simulink model "TRAS_DevDriv"  (Simulink 8.1)
settings: Solver=ode5  SolverMode=SingleTasking  StartTime=0.0  StopTime=999999  FixedStep=0.01  RelTol=1e-3  AbsTol=1e-6
undefined symbols (not defined in the file): rtdac4pcibaseaddress
settings Model: Creator=jims  LastModifiedBy=inteco  SimulationMode=external  ExtModeTrigDuration=12000
settings DataIOCC: ExternalInput=[]  InitialState=[]  LimitDataPoints=off  MaxDataPoints=5000  SaveOutput=off  SaveTime=off  SignalLoggingName=sigsOut
settings OptimizationCC: BooleanDataType=off  InitFltsAndDblsToZero=on
settings DebuggingCC: SaveWithParameterizedLinksMsg=none  SignalResolutionControl=TryResolveAllWithWarning  SolverPrmCheckMsg=none  MultiTaskDSMMsg=warning  MultiTaskCondExecSysMsg=none  IntegerOverflowMsg=none  StrictBusMsg=None
settings HardwareCC: ProdIntDivRoundTo=Zero  ProdEndianess=LittleEndian  ProdHWDeviceType=Generic->32-bit x86 compatible
settings RTWCC: SystemTargetFile=rtwin.tlc  TemplateMakefile=rtwin.tmf  Description=Real-Time Windows Target  ProcessScript=rtwin_make_rtw_hook  IncludeERTFirstTime=on  RTWCompilerOptimization=On
settings CodeAppCC: MaxIdLength=95
settings RTWinTargetCC: TargetLibSuffix=_rtwin.lib  TargetPreCompLibLocation=E:\apps_W32\MATLAB\R2013a\toolbox\rtw\targets\rtwin\lib\win32  CodeReplacementLibrary=ANSI_C  RTWinDir=E:/apps_W32/MATLAB/R2013a/toolbox/rtw/targets/rtwin  TargetArch=win32

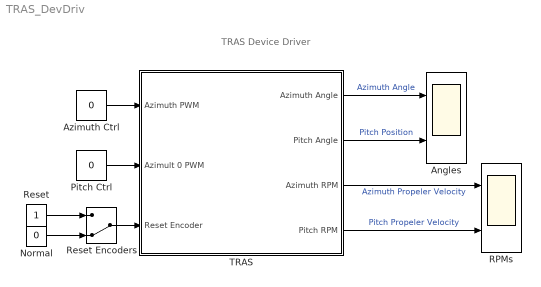
== system TRAS_DevDriv ==
  note: TRAS Device Driver
  Angles : Scope  NumInputPorts=2
      settings: TimeRange=30  YMin=-0.02~-0.1  YMax=0.0025~1  SaveName=SD1  MaxDataPoints=12000
  Azimuth Ctrl : Constant  Value=0
  Normal : Constant  Value=0
  Pitch Ctrl : Constant  Value=0
  RPMs : Scope  NumInputPorts=2
      settings: TimeRange=30  YMin=-20~-400  YMax=0~500  SaveName=SD  MaxDataPoints=12000
  Reset : Constant
  Reset Encoders : ManualSwitch  CurrentSetting=0
  TRAS : Subsystem  mask{BaseAddress=rtdac4pcibaseaddress, T0=0.01}
      mask prompts: BaseAddress "Base Address:"; T0 "Sampling Period:"
      mask Display: image(imread('TRAS.JPG'))
  wires:
  TRAS/1(Azimuth Angle) -> Angles/1  "Azimuth Angle"
  TRAS/2(Pitch Angle) -> Angles/2  "Pitch Position"
  Azimuth Ctrl/1 -> TRAS/1(Azimuth PWM)
  Pitch Ctrl/1 -> TRAS/2(Azimult 0 PWM)
  TRAS/3(Azimuth RPM) -> RPMs/1  "Azimuth Propeler Velocity"
  TRAS/4(Pitch RPM) -> RPMs/2  "Pitch Propeler Velocity"
  Normal/1 -> Reset Encoders/2
  Reset/1 -> Reset Encoders/1
  Reset Encoders/1 -> TRAS/3(Reset Encoder)

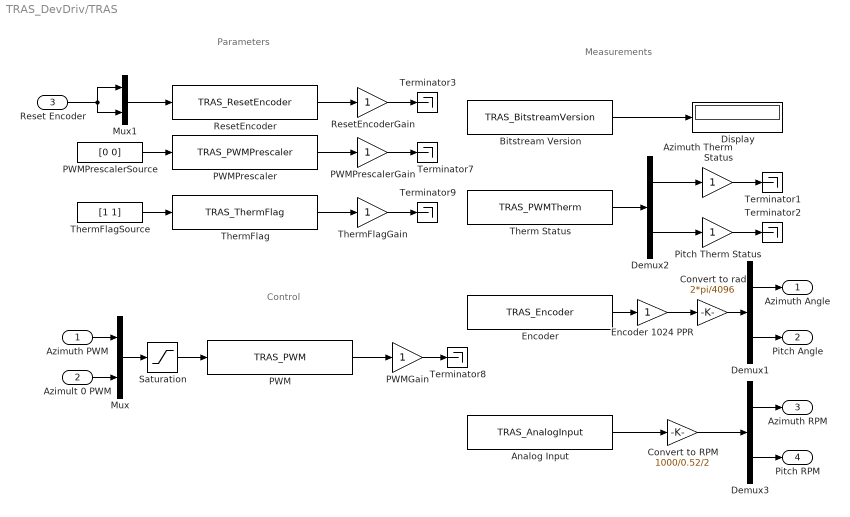
== system TRAS_DevDriv/TRAS ==
  note: Measurements
  note: Control
  note: Parameters
  Azimuth PWM : Inport
  Azimult 0 PWM : Inport  Port=2
  Reset Encoder : Inport  Port=3
  Analog Input : S-Function  FunctionName=TRAS_AnalogInput  Parameters=BaseAddress, [1 0], [1 1], T0  EnableBusSupport=off
  Azimuth Therm Status : Gain  SaturateOnIntegerOverflow=on  OutDataTypeStr=Inherit: Same as input  ParamDataTypeStr=Inherit: Same as input
  Bitstream Version : S-Function  FunctionName=TRAS_BitstreamVersion  Parameters=BaseAddress, T0  EnableBusSupport=off
  Convert to RPM : Gain  Gain=1000/0.52/2  SaturateOnIntegerOverflow=on  OutDataTypeStr=Inherit: Same as input  ParamDataTypeStr=Inherit: Same as input
  Convert to rad : Gain  Gain=2*pi/4096  SaturateOnIntegerOverflow=on  OutDataTypeStr=Inherit: Same as input  ParamDataTypeStr=Inherit: Same as input
  Demux1 : Demux  Outputs=2
  Demux2 : Demux  Outputs=2
  Demux3 : Demux  Outputs=2
  Display : Display
  Encoder : S-Function  FunctionName=TRAS_Encoder  Parameters=BaseAddress, T0  EnableBusSupport=off
  Encoder 1024 PPR : Gain  SaturateOnIntegerOverflow=on  OutDataTypeStr=Inherit: Same as input  ParamDataTypeStr=Inherit: Same as input
  Mux : Mux  Inputs=2
  Mux1 : Mux  Inputs=2
  PWM : S-Function  FunctionName=TRAS_PWM  Parameters=BaseAddress, T0  EnableBusSupport=off
  PWMGain : Gain  SaturateOnIntegerOverflow=on  OutDataTypeStr=Inherit: Same as input  ParamDataTypeStr=Inherit: Same as input
  PWMPrescaler : S-Function  FunctionName=TRAS_PWMPrescaler  Parameters=BaseAddress, T0  EnableBusSupport=off
  PWMPrescalerGain : Gain  SaturateOnIntegerOverflow=on  OutDataTypeStr=Inherit: Same as input  ParamDataTypeStr=Inherit: Same as input
  PWMPrescalerSource : Constant  Value=[0 0]
  Pitch Therm Status : Gain  SaturateOnIntegerOverflow=on  OutDataTypeStr=Inherit: Same as input  ParamDataTypeStr=Inherit: Same as input
  ResetEncoder : S-Function  FunctionName=TRAS_ResetEncoder  Parameters=BaseAddress, T0  EnableBusSupport=off
  ResetEncoderGain : Gain  SaturateOnIntegerOverflow=on  OutDataTypeStr=Inherit: Same as input  ParamDataTypeStr=Inherit: Same as input
  Saturation : Saturate  UpperLimit=1  LowerLimit=-1
  Terminator{1..3,7..9} (6 alike) : Terminator
  Therm Status : S-Function  FunctionName=TRAS_PWMTherm  Parameters=BaseAddress, T0  EnableBusSupport=off
  "ThermFlag " : S-Function  FunctionName=TRAS_ThermFlag  Parameters=BaseAddress, T0  EnableBusSupport=off
  ThermFlagGain : Gain  SaturateOnIntegerOverflow=on  OutDataTypeStr=Inherit: Same as input  ParamDataTypeStr=Inherit: Same as input
  ThermFlagSource : Constant  Value=[1 1]
  Azimuth Angle : Outport  InitialOutput=0
  Pitch Angle : Outport  Port=2  InitialOutput=0
  Azimuth RPM : Outport  Port=3  InitialOutput=0
  Pitch RPM : Outport  Port=4  InitialOutput=0
  wires:
  ThermFlagGain/1 -> Terminator9/1
  ThermFlagSource/1 -> "ThermFlag "/1
  "ThermFlag "/1 -> ThermFlagGain/1
  Convert to RPM/1 -> Demux3/1
  Reset Encoder/1 -> Mux1/2, Mux1/1
  Demux3/1 -> Azimuth RPM/1
  Demux3/2 -> Pitch RPM/1
  Analog Input/1 -> Convert to RPM/1
  Bitstream Version/1 -> Display/1
  Pitch Therm Status/1 -> Terminator2/1
  Azimuth Therm Status/1 -> Terminator1/1
  Demux2/1 -> Azimuth Therm Status/1
  Demux2/2 -> Pitch Therm Status/1
  Therm Status/1 -> Demux2/1
  Demux1/1 -> Azimuth Angle/1
  Convert to rad/1 -> Demux1/1
  Demux1/2 -> Pitch Angle/1
  Azimuth PWM/1 -> Mux/1
  Azimult 0 PWM/1 -> Mux/2
  PWMPrescalerGain/1 -> Terminator7/1
  ResetEncoderGain/1 -> Terminator3/1
  PWMPrescalerSource/1 -> PWMPrescaler/1
  Mux1/1 -> ResetEncoder/1
  PWMPrescaler/1 -> PWMPrescalerGain/1
  ResetEncoder/1 -> ResetEncoderGain/1
  PWMGain/1 -> Terminator8/1
  PWM/1 -> PWMGain/1
  Mux/1 -> Saturation/1
  Saturation/1 -> PWM/1
  Encoder/1 -> Encoder 1024 PPR/1
  Encoder 1024 PPR/1 -> Convert to rad/1
